simulink model "AC_Brushless_model"  (R2021a)
settings: Solver=ode23t  StartTime=0.0  StopTime=100
values from neighbouring files (symbols this model uses):
  B = 0.065    [AlfaRomeo_script.m]
  d = 60*10^-2    (= 0.6)    [AlfaRomeo_script.m]
  i_max = Tn/pp/eff/phi_PM    (= 974.436090226)    [AlfaRomeo_script.m]
  id_ref = [0,0,0,-phi_PM/Ls,-phi_PM/Ls,-phi_PM/Ls,     -phi_PM/Ls,-phi_PM/Ls,-phi_PM/Ls,-phi_PM/Ls,-phi_PM/Ls]    [AlfaRomeo_script.m]
  J = mass_tot*v_max^2/omega_max^2    (= 15.8)    [AlfaRomeo_script.m]
  kp_O = par_reg_speed.Kp    [AlfaRomeo_script.m]
  kp_s = par_regi.Kp    [AlfaRomeo_script.m]
  Ls = 0.8*10^-3    (= 0.0008)    [AlfaRomeo_script.m]
  phi_PM = 0.5    [AlfaRomeo_script.m]
  pp = 2    [AlfaRomeo_script.m]
  Rs = 0.1    [AlfaRomeo_script.m]
  speed_rad_sim = speed_kmh./((d/2)*tr*3.6)    [AlfaRomeo_script.m]
  speed_ref = [0, 35, 70,150,160,170,180,190,200,210,220]    [AlfaRomeo_script.m]
  Ti_O = kp_O/ki_O    [AlfaRomeo_script.m]
  Ti_s = kp_s/ki_s    [AlfaRomeo_script.m]
  tr = 1/3    (= 0.333333333333)    [AlfaRomeo_script.m]
  V_batt = 800    [AlfaRomeo_script.m]
libraries: simulink x4
settings Model: Creator=secch  LastModifiedBy=secch
settings SolverCC: ZeroCrossAlgorithm=Adaptive  AlgebraicLoopSolver=TrustRegion
settings DebuggingCC: IgnoredZcDiagnostic=none  SFMachineParentedDataDiag=warning

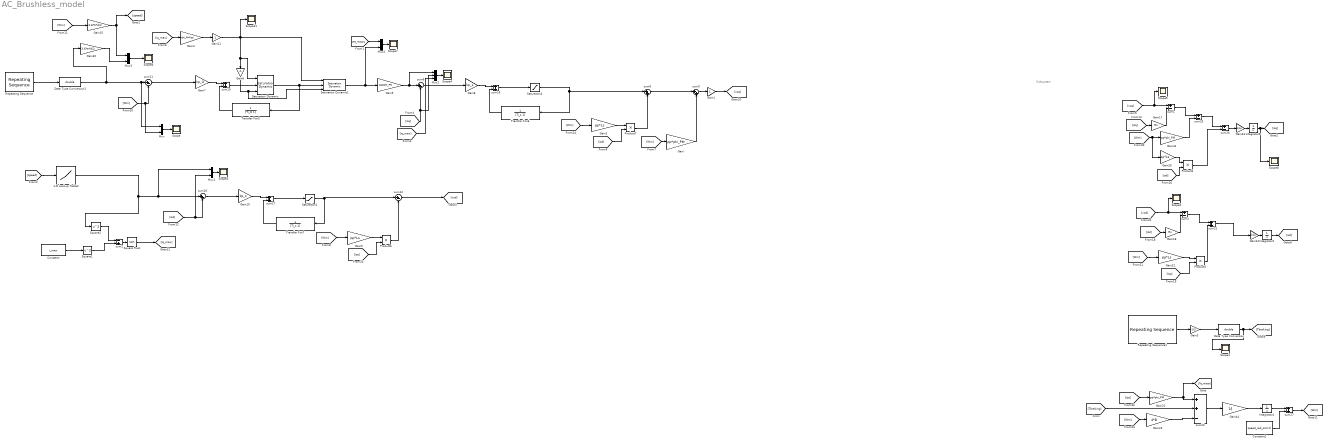
== system AC_Brushless_model ==
  note: Subsystem
  1-D Lookup Table2 : Lookup_n-D  NumberOfTableDimensions=1  BreakpointsForDimension1=speed_ref  Table=id_ref  InternalRulePriority=Speed  RndMeth=Simplest  InputSameDT=on
  Constant : Constant  Value=i_max
  Constant1 : Constant  Value=speed_rad_sim(1)
  Data Type Conversion : DataTypeConversion  OutDataTypeStr=double
  Data Type Conversion1 : DataTypeConversion  OutDataTypeStr=double
  Gain : Gain  Gain=pp*phi_PM
  Gain1 : Gain
  Gain10 : Gain  Gain=kp_s
  Gain11 : Gain
  Gain15 : Gain  Gain=3.6*tr*d/2
  Gain17 : Gain  Gain=Rs
  Gain18 : Gain  Gain=Rs
  Gain{2,5,22,26} (4 alike) : Gain  Gain=pp*Ls
  Gain21 : Gain  Gain=pp*phi_PM
  Gain23 : Gain  Gain=4*B
  Gain24 : Gain  Gain=1/Ls
  Gain3 : Gain  Gain=1/3
  Gain30 : Gain  Gain=3.6*tr*d/2
  Gain4 : Gain  Gain=phi_PM*pp
  Gain42 : Gain  Gain=pp*phi_PM
  Gain43 : Gain  Gain=1/Ls
  Gain44 : Gain  Gain=1/J
  Gain6 : Gain  Gain=-1
  Gain7 : Gain  Gain=kp_O
  Gain8 : Gain  Gain=kp_s
  Gain9 : Gain  Gain=1/pp/phi_PM
  Integrator2 : Integrator
  Integrator3 : Integrator
  Integrator4 : Integrator
  Mux{,1,3..4} (4 alike) : Mux  Inputs=2
  Mux2 : Mux  Inputs=3
  Product{2,5..7} (4 alike) : Product
  Repeating Sequence : simulink/Sources/Repeating Sequence  rep_seq_t=time  rep_seq_y=speed_rad_sim
  Repeating Sequence1 : simulink/Sources/Repeating Sequence  rep_seq_t=time(2:end)  rep_seq_y=T_braking(2:end)
  Saturation Dynamic : simulink/Discontinuities/Saturation Dynamic  OutMin=[]  OutMax=[]  OutDataTypeStr=Inherit: Same as second input  OutDataType=fixdt(1, 16)  OutScaling=2^-10  DoSatur=off
  Saturation Dynamic1 : simulink/Discontinuities/Saturation Dynamic  OutMin=[]  OutMax=[]  OutDataTypeStr=Inherit: Same as second input  OutDataType=fixdt(1, 16)  OutScaling=2^-10  DoSatur=off
  Saturation1 : Saturate  UpperLimit=V_batt  LowerLimit=-V_batt
  Saturation4 : Saturate  UpperLimit=V_batt  LowerLimit=-V_batt
  Scope{,1..8,21} (10 alike) : Scope
  Square Root : Sqrt  SaturateOnIntegerOverflow=on
  Square1 : Math  Operator=square  SaturateOnIntegerOverflow=on
  Square2 : Math  Operator=square  SaturateOnIntegerOverflow=on
  Transfer Fcn5 : TransferFcn  Denominator=[Ti_O 1]
  Transfer Fcn6 : TransferFcn  Denominator=[Ti_s 1]
  Transfer Fcn7 : TransferFcn  Denominator=[Ti_s 1]
  sum{1,3,25..26} (4 alike) : Sum  Inputs=+-
  sum{6,10..12} (4 alike) : Sum  Inputs=|+-
  sum{15..17,21,27} (5 alike) : Sum
  sum2 : Sum  Inputs=-+
  sum22 : Sum  Inputs=++-
  sum8 : Sum  Inputs=|++
  sum9 : Sum  Inputs=|++
  wires:
  sum9/1 -> Gain1/1
  Product6/1 -> sum12/2
  Saturation1/1 -> Transfer Fcn7/1, sum12/1
  sum8/1 -> sum9/1
  Gain/1 -> sum9/2
  Saturation4/1 -> sum8/1, Transfer Fcn6/1
  Gain9/1 -> Mux2/1, sum6/1
  Saturation Dynamic/1 -> Saturation Dynamic1/2, Transfer Fcn5/1
  [Wm] -> Mux/2, sum11/2
  [isq] -> Mux2/2, sum6/2
  Gain7/1 -> sum15/1
  sum15/1 -> Saturation Dynamic/2
  sum11/1 -> Gain7/1
  Gain6/1 -> Saturation Dynamic1/3, Saturation Dynamic/3
  Transfer Fcn5/1 -> sum15/2
  Transfer Fcn6/1 -> sum16/2
  sum6/1 -> Gain8/1
  sum16/1 -> Saturation4/1
  Gain8/1 -> sum16/1
  Transfer Fcn7/1 -> sum17/2
  sum10/1 -> Gain10/1
  sum17/1 -> Saturation1/1
  Gain10/1 -> sum17/1
  [speed] -> 1-D Lookup Table2/1
  Gain1/1 -> [vsq]
  [Wm] -> Gain15/1
  Gain15/1 -> [speed], Mux3/1
  [isq] -> Gain17/1
  sum1/1 -> sum25/1
  Gain17/1 -> sum1/2
  [vsq] -> Scope5/1, sum1/1
  [isd] -> Mux1/2, sum10/2
  Mux/1 -> Scope/1
  Repeating Sequence/1 -> Data Type Conversion1/1
  Mux3/1 -> Scope6/1
  Gain30/1 -> Mux3/2
  [Wm] -> Gain26/1, Gain42/1
  Gain42/1 -> sum25/2
  Gain26/1 -> Product2/1
  [isd] -> Product2/2
  Product2/1 -> sum26/2
  sum25/1 -> sum26/1
  sum26/1 -> Gain43/1
  Gain43/1 -> Integrator2/1
  Integrator2/1 -> Scope8/1, [isq]
  Integrator3/1 -> [isd]
  Gain24/1 -> Integrator3/1
  sum21/1 -> Gain24/1
  [Wm] -> Gain22/1
  [vsd] -> sum3/1, Scope2/1
  Gain18/1 -> sum3/2
  sum3/1 -> sum21/1
  [isd] -> Gain18/1
  Gain22/1 -> Product5/1
  [isq] -> Product5/2
  Product5/1 -> sum21/2
  [isq] -> Gain21/1
  [Wm] -> Gain23/1
  Gain23/1 -> sum22/3
  Gain21/1 -> [Te_motor], sum22/1
  Repeating Sequence1/1 -> Gain3/1
  sum22/1 -> Gain44/1
  Gain44/1 -> Integrator4/1
  Integrator4/1 -> sum27/1
  Constant1/1 -> sum27/2
  sum27/1 -> [Wm]
  [Wm] -> Gain5/1
  Gain5/1 -> Product6/1
  [isq] -> Product6/2
  sum12/1 -> [vsd]
  Constant/1 -> Square1/1
  Square2/1 -> sum2/1
  Square1/1 -> sum2/2
  sum2/1 -> Square Root/1
  Square Root/1 -> [iq_max]
  [Wm] -> Gain2/1
  [isd] -> Product7/2
  Gain2/1 -> Product7/1
  Product7/1 -> sum8/2
  [Wm] -> Gain/1
  Saturation Dynamic1/1 -> Mux4/2, Gain9/1
  Data Type Conversion/1 -> Scope1/1, [Tbraking]
  Data Type Conversion1/1 -> Gain30/1, Mux/1, sum11/1
  [Tbraking] -> sum22/2
  Mux1/1 -> Scope3/1
  Mux2/1 -> Scope4/1
  Mux4/1 -> Scope7/1
  [Te_motor] -> Mux4/1
  Gain4/1 -> Gain11/1
  1-D Lookup Table2/1 -> Mux1/1, sum10/1, Square2/1
  [iq_max] -> Gain4/1
  Gain3/1 -> Data Type Conversion/1
  Gain11/1 -> Saturation Dynamic/1, Gain6/1, Scope21/1, Saturation Dynamic1/1
  [iq_max] -> Mux2/3
